simulink model "simulation1"  (R2021b)
settings: Solver=ode15s  StartTime=0.0  StopTime=40.0  RelTol=1e-3
values from neighbouring files (symbols this model uses):
  a = [-2.0 2.0 ... (first row only)    [init.m]
  A_p = [0  1   0  0   0  0 ... (first row only)    [init.m]
  b = [-0.05  0.05 ... (first row only)    [init.m]
  B_p = [0     0     0 ... (first row only)    [init.m]
  B_p_d = [-0.2  0    0 ... (first row only)    [init.m]
  epsilon_1 = 1e-17    [init.m]
  epsilon_2 = 1e-17    [init.m]
  f_0 = 20*ones(4,1)    [init.m]
  f_max = 200*ones(m,1)    [init.m]
  f_min = 10*ones(m,1)    [init.m]
  f_ref = 0.5*(f_min+f_max)    [init.m]
  k_spring = diag(2000*ones(m,1))    [init.m]
  k_spring_inv = inv(k_spring)    [init.m]
  l = inverseKinematics(a, b, x, m)    [init.m]
  m = 4    [init.m]
  tau = 1e-6    (= 1e-06)    [init.m]
  x = [r; 0]    [init.m]
  x_0 = [x(1); 0; x(2); 0; x(3);0]    [init.m]
  x_d = [0.0;0.5;0]    [init.m]
  xi = 2    [init.m]
libraries: simulink x2, simulink_extras x1
settings Model: Creator=Sølve  LastModifiedBy=Sølve

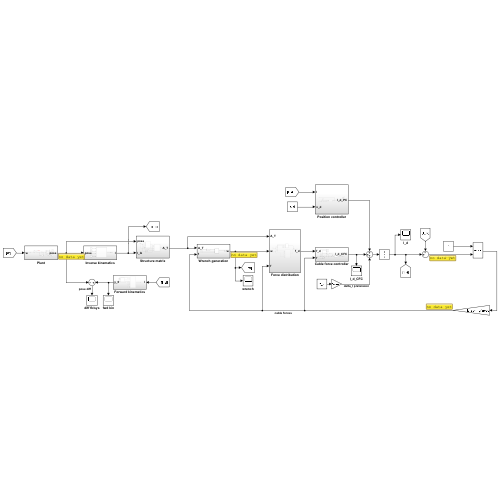
[thumbnail: Simulink's stored preview of the top-level diagram]
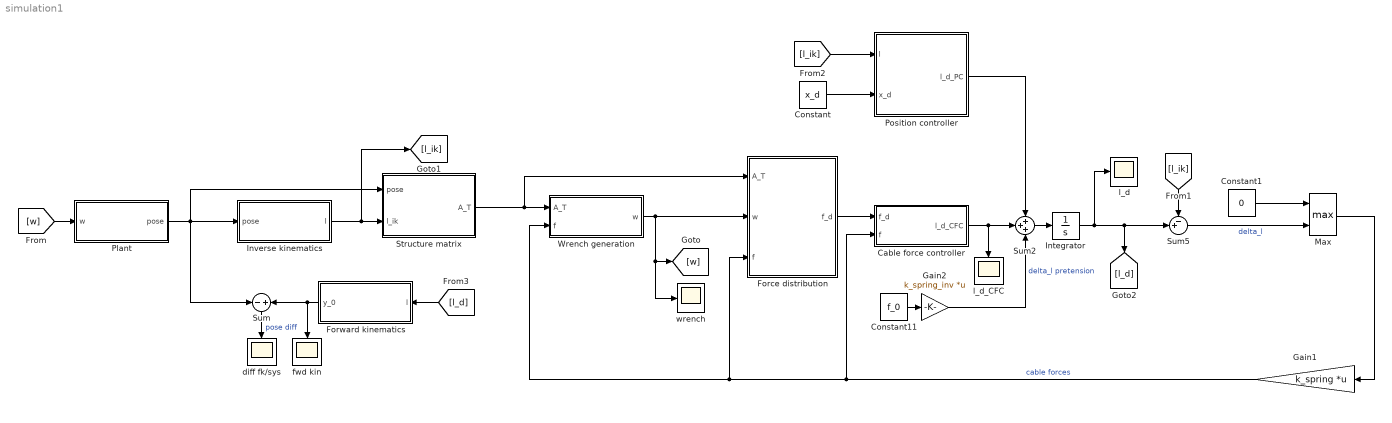
== system simulation1 ==
  Cable force controller : Subsystem
  Constant : Constant  Value=x_d
  Constant1 : Constant  Value=0
  Constant11 : Constant  Value=f_0
  Force distribution : Subsystem
  Forward kinematics : Subsystem
  Gain1 : Gain  Gain=k_spring  Multiplication=Matrix(K*u) (u vector)
  Gain2 : Gain  Gain=k_spring_inv  Multiplication=Matrix(K*u) (u vector)
  Integrator : Integrator  InitialCondition=l
  Inverse kinematics : Subsystem
  Max : MinMax  Function=max  Inputs=2
  Plant : Subsystem
  Position controller : Subsystem
  Structure matrix : Subsystem
  Sum : Sum  Inputs=-|+
  Sum2 : Sum  Inputs=+++
  Sum5 : Sum  Inputs=-+|
  Wrench generation : Subsystem
  diff fk/sys : Scope
  fwd kin : Scope
  l_d : Scope
  l_d_CFC : Scope
  wrench : Scope
  wires:
  Inverse kinematics/1(l) -> [l_ik], Structure matrix/2(l_ik)
  Structure matrix/1(A_T) -> Force distribution/1(A_T), Wrench generation/1(A_T)
  Force distribution/1(f_d) -> Cable force controller/1(f_d)
  Cable force controller/1(l_d_CFC) -> Sum2/2, l_d_CFC/1
  Sum2/1 -> Integrator/1
  Integrator/1 -> Sum5/2, [l_d], l_d/1
  Constant1/1 -> Max/1
  Sum5/1 -> Max/2  "delta_l"
  Max/1 -> Gain1/1
  Gain1/1 -> Wrench generation/2(f), Force distribution/3(f), Cable force controller/2(f)  "cable forces"
  Wrench generation/1(w) -> Force distribution/2(w), [w], wrench/1
  Constant11/1 -> Gain2/1
  Gain2/1 -> Sum2/3  "delta_l pretension"
  Forward kinematics/1(y_0) -> Sum/2, fwd kin/1
  Sum/1 -> diff fk/sys/1  "pose diff"
  [w] -> Plant/1(w)
  [l_ik] -> Sum5/1
  [l_d] -> Forward kinematics/1(l)
  Plant/1(pose) -> Inverse kinematics/1(pose), Sum/1, Structure matrix/1(pose)
  [l_ik] -> Position controller/1(l)
  Constant/1 -> Position controller/2(x_d)
  Position controller/1(l_d_PC) -> Sum2/1

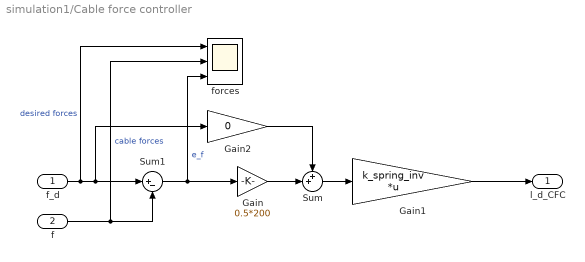
== system simulation1/Cable force controller ==
  f_d : Inport
  f : Inport  Port=2
  Gain : Gain  Gain=0.5*200
  Gain1 : Gain  Gain=k_spring_inv  Multiplication=Matrix(K*u) (u vector)
  Gain2 : Gain  Gain=0
  Sum : Sum  Inputs=++|
  Sum1 : Sum  Inputs=|+-
  forces : Scope  NumInputPorts=3
  l_d_CFC : Outport
  wires:
  Gain/1 -> Sum/2
  f_d/1 -> forces/1, Sum1/1, Gain2/1  "desired forces"
  Gain1/1 -> l_d_CFC/1
  Sum/1 -> Gain1/1
  Sum1/1 -> forces/3, Gain/1  "e_f"
  f/1 -> forces/2, Sum1/2  "cable forces"
  Gain2/1 -> Sum/1

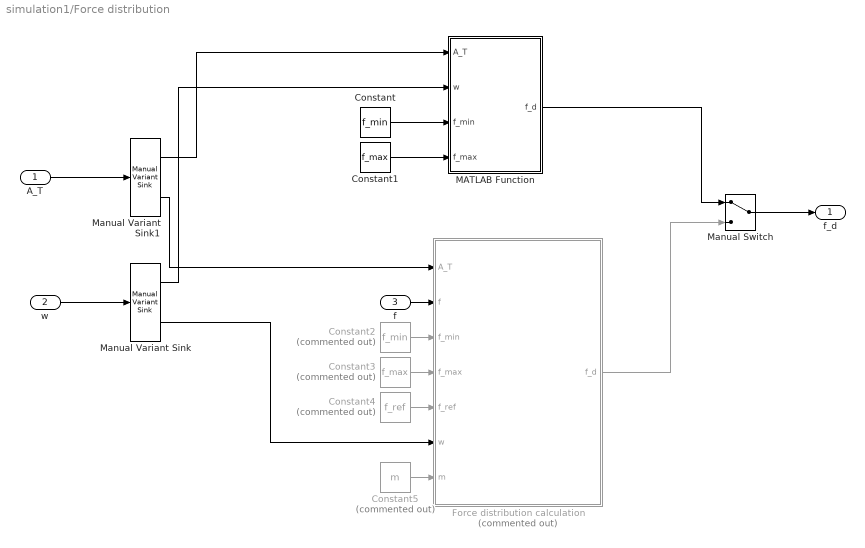
== system simulation1/Force distribution ==
  A_T : Inport
  w : Inport  Port=2
  f : Inport  Port=3
  Constant : Constant  Value=f_min
  Constant1 : Constant  Value=f_max
  Constant2 : Constant  Commented=on  Value=f_min
  Constant3 : Constant  Commented=on  Value=f_max
  Constant4 : Constant  Commented=on  Value=f_ref
  Constant5 : Constant  Commented=on  Value=m
  Force distribution calculation : MATLAB Function  Commented=on  TreatAsAtomicUnit=on
  MATLAB Function : MATLAB Function  TreatAsAtomicUnit=on
  Manual Variant Sink : simulink/Signal Routing/Manual Variant Sink  NumChoices=2  LabelModeActiveChoice=V_1
  Manual Variant Sink1 : simulink/Signal Routing/Manual Variant Sink  NumChoices=2  LabelModeActiveChoice=V_1
  Manual Switch : ManualSwitch
  f_d : Outport
  wires:
  A_T/1 -> Manual Variant Sink1/1
  MATLAB Function/1(f_d) -> Manual Switch/1
  Constant1/1 -> MATLAB Function/4(f_max)
  Constant/1 -> MATLAB Function/3(f_min)
  w/1 -> Manual Variant Sink/1
  Force distribution calculation/1(f_d) -> Manual Switch/2
  Constant5/1 -> Force distribution calculation/7(m)
  Constant2/1 -> Force distribution calculation/3(f_min)
  Constant3/1 -> Force distribution calculation/4(f_max)
  Manual Variant Sink/2 -> Force distribution calculation/6(w)
  f/1 -> Force distribution calculation/2(f)
  Constant4/1 -> Force distribution calculation/5(f_ref)
  Manual Variant Sink1/2 -> Force distribution calculation/1(A_T)
  Manual Variant Sink/1 -> MATLAB Function/2(w)
  Manual Variant Sink1/1 -> MATLAB Function/1(A_T)
  Manual Switch/1 -> f_d/1

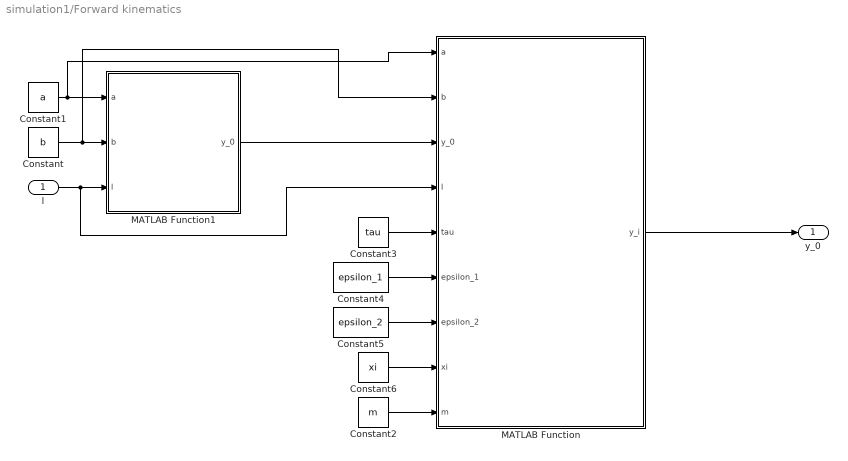
== system simulation1/Forward kinematics ==
  l : Inport
  Constant : Constant  Value=b
  Constant1 : Constant  Value=a
  Constant2 : Constant  Value=m
  Constant3 : Constant  Value=tau
  Constant4 : Constant  Value=epsilon_1
  Constant5 : Constant  Value=epsilon_2
  Constant6 : Constant  Value=xi
  MATLAB Function : MATLAB Function  TreatAsAtomicUnit=on
  MATLAB Function1 : MATLAB Function  TreatAsAtomicUnit=on
  y_0 : Outport
  wires:
  l/1 -> MATLAB Function1/3(l), MATLAB Function/4(l)
  Constant/1 -> MATLAB Function1/2(b), MATLAB Function/2(b)
  Constant1/1 -> MATLAB Function1/1(a), MATLAB Function/1(a)
  MATLAB Function1/1(y_0) -> MATLAB Function/3(y_0)
  Constant2/1 -> MATLAB Function/9(m)
  MATLAB Function/1(y_i) -> y_0/1
  Constant3/1 -> MATLAB Function/5(tau)
  Constant5/1 -> MATLAB Function/7(epsilon_2)
  Constant4/1 -> MATLAB Function/6(epsilon_1)
  Constant6/1 -> MATLAB Function/8(xi)

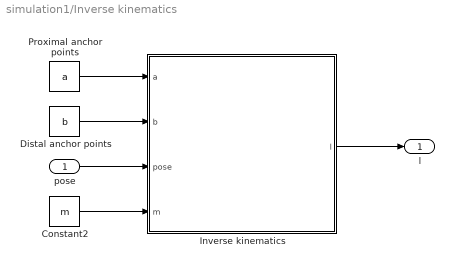
== system simulation1/Inverse kinematics ==
  pose : Inport
  Constant2 : Constant  Value=m
  Distal anchor points : Constant  Value=b
  Inverse kinematics : MATLAB Function  TreatAsAtomicUnit=on
  Proximal anchor points : Constant  Value=a
  l : Outport
  wires:
  pose/1 -> Inverse kinematics/3(pose)
  Constant2/1 -> Inverse kinematics/4(m)
  Distal anchor points/1 -> Inverse kinematics/2(b)
  Proximal anchor points/1 -> Inverse kinematics/1(a)
  Inverse kinematics/1(l) -> l/1

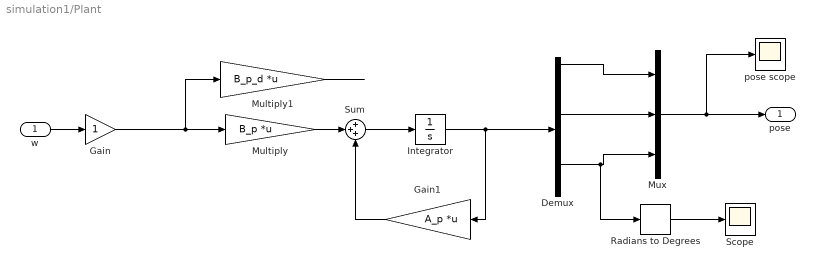
== system simulation1/Plant ==
  w : Inport
  Demux : Demux  Outputs=6
  Gain : Gain
  Gain1 : Gain  Gain=A_p  Multiplication=Matrix(K*u) (u vector)
  Integrator : Integrator  InitialCondition=x_0
  Multiply : Gain  Gain=B_p  Multiplication=Matrix(K*u) (u vector)
  Multiply1 : Gain  Gain=B_p_d  Multiplication=Matrix(K*u) (u vector)
  Mux : Mux  Inputs=3
  Radians to Degrees : simulink_extras/Transformations/Radians to Degrees
  Scope : Scope
  Sum : Sum  Inputs=+++
  pose scope : Scope
  pose : Outport
  wires:
  w/1 -> Gain/1
  Gain/1 -> Multiply1/1, Multiply/1
  Multiply/1 -> Sum/2
  Sum/1 -> Integrator/1
  Gain1/1 -> Sum/3
  Integrator/1 -> Demux/1, Gain1/1
  Demux/1 -> Mux/1
  Demux/3 -> Mux/2
  Demux/5 -> Radians to Degrees/1, Mux/3
  Mux/1 -> pose scope/1, pose/1
  Multiply1/1 -> ?
  Radians to Degrees/1 -> Scope/1

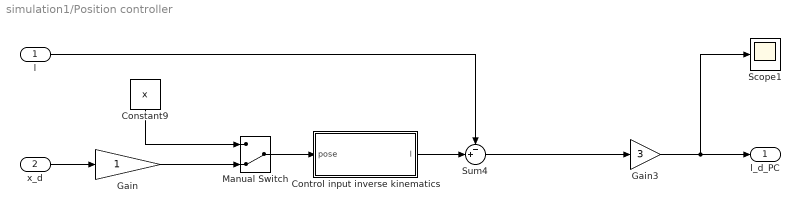
== system simulation1/Position controller ==
  l : Inport
  x_d : Inport  Port=2
  Constant9 : Constant  Value=x
  Control input inverse kinematics : Subsystem
  Gain : Gain
  Gain3 : Gain  Gain=3
  Manual Switch : ManualSwitch  CurrentSetting=0
  Scope1 : Scope
  Sum4 : Sum  Inputs=-+|
  l_d_PC : Outport
  wires:
  Control input inverse kinematics/1(l) -> Sum4/2
  Sum4/1 -> Gain3/1
  Gain/1 -> Manual Switch/2
  Gain3/1 -> Scope1/1, l_d_PC/1
  x_d/1 -> Gain/1
  Constant9/1 -> Manual Switch/1
  Manual Switch/1 -> Control input inverse kinematics/1(pose)
  l/1 -> Sum4/1

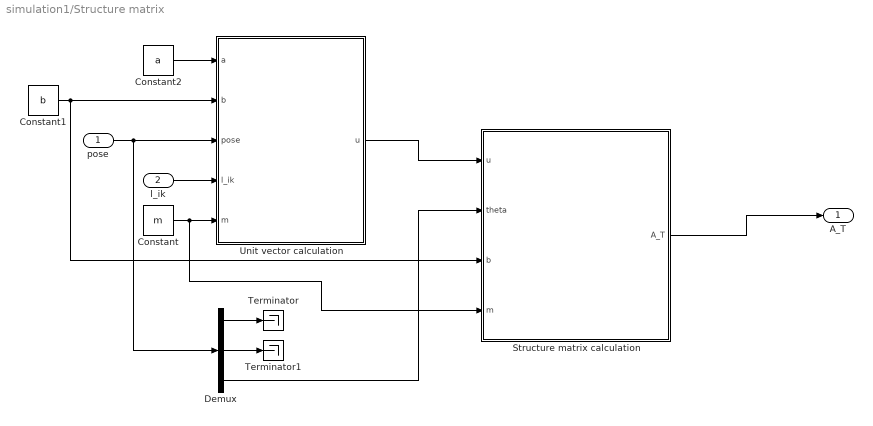
== system simulation1/Structure matrix ==
  pose : Inport
  l_ik : Inport  Port=2
  Constant : Constant  Value=m
  Constant1 : Constant  Value=b
  Constant2 : Constant  Value=a
  Demux : Demux  Outputs=3
  Structure matrix calculation : MATLAB Function  TreatAsAtomicUnit=on
  Terminator : Terminator
  Terminator1 : Terminator
  Unit vector calculation : MATLAB Function  TreatAsAtomicUnit=on
  A_T : Outport
  wires:
  l_ik/1 -> Unit vector calculation/4(l_ik)
  pose/1 -> Demux/1, Unit vector calculation/3(pose)
  Constant/1 -> Structure matrix calculation/4(m), Unit vector calculation/5(m)
  Constant2/1 -> Unit vector calculation/1(a)
  Constant1/1 -> Structure matrix calculation/3(b), Unit vector calculation/2(b)
  Unit vector calculation/1(u) -> Structure matrix calculation/1(u)
  Structure matrix calculation/1(A_T) -> A_T/1
  Demux/3 -> Structure matrix calculation/2(theta)
  Demux/2 -> Terminator1/1
  Demux/1 -> Terminator/1

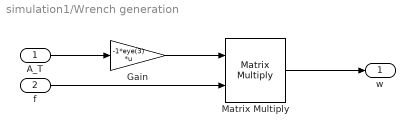
== system simulation1/Wrench generation ==
  A_T : Inport
  f : Inport  Port=2
  Gain : Gain  Gain=-1*eye(3)  Multiplication=Matrix(K*u)
  Matrix Multiply : Product  Multiplication=Matrix(*)
  w : Outport
  wires:
  A_T/1 -> Gain/1
  f/1 -> Matrix Multiply/2
  Gain/1 -> Matrix Multiply/1
  Matrix Multiply/1 -> w/1

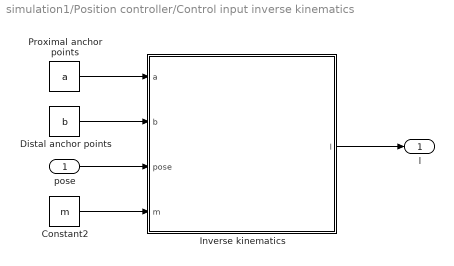
== system simulation1/Position controller/Control input inverse kinematics ==
  pose : Inport
  Constant2 : Constant  Value=m
  Distal anchor points : Constant  Value=b
  Inverse kinematics : MATLAB Function  TreatAsAtomicUnit=on
  Proximal anchor points : Constant  Value=a
  l : Outport
  wires:
  Inverse kinematics/1(l) -> l/1
  Proximal anchor points/1 -> Inverse kinematics/1(a)
  Distal anchor points/1 -> Inverse kinematics/2(b)
  Constant2/1 -> Inverse kinematics/4(m)
  pose/1 -> Inverse kinematics/3(pose)

== matlab function simulation1/Structure matrix/Unit vector calculation ==
  data: a input; u output; b input; pose input; l_ik input; m input
function u = calculateCableUnitVectors(a, b, pose, l_ik, m)
    r = pose(1:2);
    theta = pose(3);
    l = a - r - R_z(theta)*b;
    u = zeros(2,4);
    for i=1:m
        u(:,i) = l(:,i)/l_ik(i);
    end
end

function R = R_z(theta)
    R = [cos(theta) -sin(theta);
         sin(theta)  cos(theta)];
end

== matlab function simulation1/Inverse kinematics/Inverse kinematics ==
  data: a input; l output; b input; pose input; m input
function l = inverseKinematics(a, b, pose, m)
    x     = pose(1);
    y     = pose(2);
    theta = pose(3);

    l = zeros(4,1);
    for i=1:m
        l(i) = norm(a(:,i)-[x;y]-R_z(theta)*b(:,i),2);
    end
end


function R = R_z(theta)
    R = [cos(theta) -sin(theta);
         sin(theta)  cos(theta)];
end

== matlab function simulation1/Structure matrix/Structure matrix calculation ==
  data: u input; A_T output; theta input; b input; m input
function A_T = calculateStructureMatrix(u, theta, b, m)
    crossProd = zeros(3, 4);
    for i=1:m
        crossProd(:,i) = cross([0;R_z(theta)*b(:,i);], [0;u(:,i)]);
    end
    A_T = [u; -crossProd(1,:)];
end

function R = R_z(theta)
    R = [cos(theta) -sin(theta);
         sin(theta)  cos(theta)];
end

== matlab function simulation1/Force distribution/Force distribution calculation ==
  data: A_T input; f input; f_d output; f_min input; f_max input; f_ref input; w input; m input
function f_d = forceQP(A_T, f, f_min, f_max, f_ref, w, m)
function f_d = forceQP(A_T, f, f_min, f_max, f_ref, w, m)
function f_d = forceQP(A_T, f, f_min, f_max, f_ref, w, m)
    coder.extrinsic('quadprog');
    f_d = zeros(4,1);
    A_T
    f_min
    f_max
    f_ref
    w
    f_d = quadprog(eye(m),-f_ref,[],[],A_T, -w,f_min,f_max, f);

== matlab function simulation1/Position controller/Control input inverse kinematics/Inverse kinematics ==
  data: a input; l output; b input; pose input; m input
function l = inverseKinematics(a, b, pose, m)
    x     = pose(1);
    y     = pose(2);
    theta = pose(3);

    l = zeros(4,1);
    for i=1:m
        l(i) = norm(a(:,i)-[x;y]-R_z(theta)*b(:,i),2);
    end
end


function R = R_z(theta)
    R = [cos(theta) -sin(theta);
         sin(theta)  cos(theta)];
end

== matlab function simulation1/Force distribution/MATLAB Function ==
  data: A_T input; f_d output; w input; f_min input; f_max input
function f_d = fcn(A_T, w, f_min, f_max)
A_T_Pinv = pinv(A_T);
f_ref = (f_min + f_max)/2;
f_d = f_ref - A_T_Pinv*(w + A_T*f_ref);
%  = u;

== matlab function simulation1/Forward kinematics/MATLAB Function ==
  data: a input; y_i output; b input; y_0 input; l input; tau input; epsilon_1 input; epsilon_2 input; xi input; m input
function y_i = MarLevPoseEstimation(a, b, y_0, l, ...
                                    tau, epsilon_1, epsilon_2, xi, ...
                                    m)
    y_i = y_0;
    
    m = size(a, 2);
    
    J = Jacobian(a, b, y_i, l, 1);
    A = J.'*J;
    phi = getPhi(a, b, y_i, l, m);
    g = J.'*phi;
    
    
%     tau       = 1e-6;
    mu        = tau*max(diag(A));
%     epsilon_1 = 1e-17;
%     epsilon_2 = 1e-17;
%     xi        = 2;
    
    iter = 0;
    max_iter = 100;
    
    stop = false;
    while ~stop && iter < max_iter
        iter = iter+1;
    
        h = (A + mu*eye(3))\(-g);
        
        if norm(h,2) <= epsilon_2*(norm(y_i,2)+epsilon_2)
            stop = true;
%             disp(epsilon_2*(norm(y_i,2)+epsilon_2));
%             disp('Stopping algorithm')
        else
            y_new = y_i + h;
    
            % Gain ratio
            Phi = 0.5*(phi.')*phi;
            phi_x_plus_h = getPhi(a, b, y_new, l, m);
            
            Phi_x_plus_h = 0.5*(phi_x_plus_h.')*phi_x_plus_h;
            rho = (Phi - Phi_x_plus_h)/(0.5*(h.')*(mu*h - g));
    
            if rho > 0
                y_i = y_new;
                J = Jacobian(a, b, y_i, l, 1);
                A = J.'*J;
                phi = getPhi(a, b, y_i, l, m);
                g = J.'*phi;
                cond = norm(g,2) < epsilon_1;
                if cond
%                     disp('Stopping algorithm 2')
                    stop = cond;
                end
                mu = mu*max([1/3, 1-(2*rho-1)^3]);
                xi = 2;
            else
                mu = mu*xi;
                xi = 2*xi;
            end
        end
    end
end

function phi = getPhi(a, b, y, l, k_spring, m)
    phi = zeros(4,1);
    for i = 1:size(phi,1)
        phi(i) = nuSquared(a(:,i), b(:,i), y(:), l(i), k_spring);
    end
end

function nuSquared = nuSquared(a, b, y, l, k_spring)
    nuSquared = ...
        k_spring*( ...
              (a(1) - y(1) - b(1)*cos(y(3)) + b(2)*sin(y(3)))^2 ...
            + (y(2) - a(2) + b(2)*cos(y(3)) + b(1)*sin(y(3)))^2 ...
            - l^2 ...
        )^2;
end


function J = Jacobian(a, b, yvec, lvec, k_spring)
    n = size(yvec,1);
    m = size(a,2);

    J = zeros(m,n);
    for i=1:m

        ax = a(1,i);
        ay = a(2,i);
        bx = b(1,i);
        by = b(2,i);
        x     = yvec(1);
        y     = yvec(2);
        theta = yvec(3);
        l = lvec(i);

        k_spring = 1;
        J_x = ...
        -2*k_spring*(    (ax - x - bx*cos(theta) + by*sin(theta))^2        ...
                     +   (y - ay + by*cos(theta) + bx*sin(theta))^2 - l^2) ...
                     * 2*(ax - x - bx*cos(theta) + by*sin(theta));
     
        J_y = ...
         2*k_spring*(   (ax - x - bx*cos(theta) + by*sin(theta))^2         ...
                     +  (y - ay + by*cos(theta) + bx*sin(theta))^2 - l^2)  ...
                     *2*(y - ay + by*cos(theta) + bx*sin(theta));
     
        J_theta = ...
         2*k_spring*(  2*(by*cos(theta) + bx*sin(theta))                   ...
                        *(ax - x - bx*cos(theta) + by*sin(theta))          ...
                     + 2*(bx*cos(theta) - by*sin(theta))                   ...
                        *(y - ay + by*cos(theta) + bx*sin(theta)))         ...
                       *((ax - x - bx*cos(theta) + by*sin(theta))^2        ...
                       + (y - ay + by*cos(theta) + bx*sin(theta))^2 - l^2);
        J(i,:) = [J_x J_y J_theta];
    end
end

== matlab function simulation1/Forward kinematics/MATLAB Function1 ==
  data: a input; y_0 output; b input; l input
function y_0 = initialPoseEstimate(a, b, l)
    m = size(a,2);
    r_low_i  = zeros(2, m);
    r_high_i = zeros(2, m);
    
    for i=1:m
        r_low_i(:, i)  = ...
            a(:,i) - (l(i) + norm(b(:,i), 2))*[1;1];
        r_high_i(:, i) = ...
            a(:,i) + (l(i) + norm(b(:,i), 2))*[1;1];
    end
    
    r_low = [max(r_low_i(1,:)); 
             max(r_low_i(2,:))];
    
    r_high = [min(r_high_i(1,:));
              min(r_high_i(2,:));];
    
    r_0 = [0.5*(r_low(1) + r_high(1)); 
           0.5*(r_low(2) + r_high(2))];
    y_0 = [r_0; 0.0];
end
